simulink model "State_Feedback"  (R2018b)
settings: Solver=VariableStepAuto  StartTime=0.0  StopTime=5  RelTol=1e-3
values from neighbouring files (symbols this model uses):
  A = zeros(5,5)    [kalmanfilter.m]    (also in model_2017.m = [[0  0   0   0                0             0   1           ; model_rough.m; model_v2.m = [[0  0   0   0                0             0   1           ; model_v3.m = [[0  0   0   0                0             0   1           )
  B = zeros(5,6)    [kalmanfilter.m]    (also in model_2017.m = [[0      0      0      0     ];                        [0   ; model_rough.m; model_v2.m = [[0      0      0      0     ];                        [0   ; model_v3.m = [[0      0      0      0      0      0             ];       )
  C = eye(5)    [kalmanfilter.m]    (also in model_2017.m = [[0  0   0   0   0   0   1   0   0   0   0   0]; model_rough.m; model_v2.m = [[0  0   0   0   0   0   1   0   0   0   0   0]; model_v3.m = [[0  0   0   0   0   0   1   0   0   0   0   0])
  K = []    [kalmanfilter.m]    (also in model_rough.m = place(A, B, polevec))
settings Model: Creator=Rishabh  LastModifiedBy=Rishabh

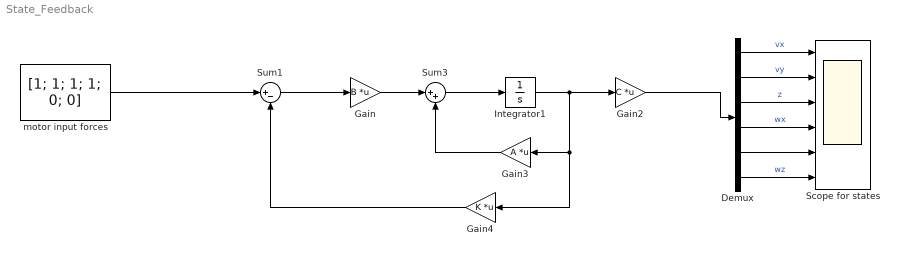
== system State_Feedback ==
  Demux : Demux  Outputs=6
  Gain : Gain  Gain=B  Multiplication=Matrix(K*u)
  Gain2 : Gain  Gain=C  Multiplication=Matrix(K*u)
  Gain3 : Gain  Gain=A  Multiplication=Matrix(K*u)
  Gain4 : Gain  Gain=K  Multiplication=Matrix(K*u)
  Integrator1 : Integrator
  Scope for states : Scope  NumInputPorts=6
  Sum1 : Sum  Inputs=|+-
  Sum3 : Sum  Inputs=|++
  motor input forces : Constant  Value=[1; 1; 1; 1; 0; 0]  VectorParams1D=off
  wires:
  motor input forces/1 -> Sum1/1
  Sum1/1 -> Gain/1
  Gain/1 -> Sum3/1
  Sum3/1 -> Integrator1/1
  Integrator1/1 -> Gain4/1, Gain3/1, Gain2/1
  Gain2/1 -> Demux/1
  Demux/1 -> Scope for states/1  "vx"
  Demux/2 -> Scope for states/2  "vy"
  Demux/3 -> Scope for states/3  "z"
  Demux/4 -> Scope for states/4  "wx"
  Demux/5 -> Scope for states/5
  Demux/6 -> Scope for states/6  "wz"
  Gain3/1 -> Sum3/2
  Gain4/1 -> Sum1/2
